simulink model "basic_pid_impedance"  (R2015a)
settings: Solver=ode45  StartTime=0.0  StopTime=10.0  RelTol=1e-3
values from neighbouring files (symbols this model uses):
  pid_imp_Kd = 2    [parameters.m]
  pid_imp_Kp = 40    [parameters.m]
  tau_max = 5    [parameters.m]
undefined symbols (not defined in the file or in its folder): pid
libraries: simulink x1
settings Model: Creator=preston  LastModifiedBy=Nathan

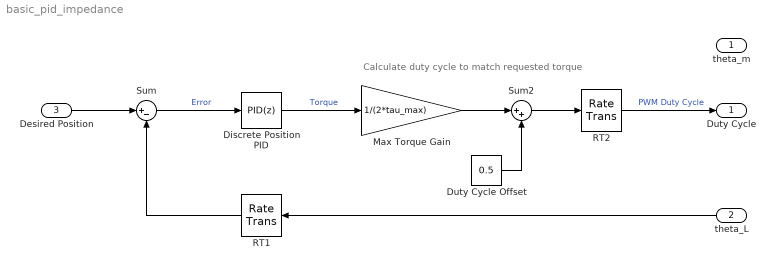
== system basic_pid_impedance ==
  note: Calculate duty cycle to match requested torque
  theta_m : Inport
  theta_L : Inport  Port=2
  Desired Position : Inport  Port=3
  Discrete Position PID : simulink/Continuous/PID Controller  Controller=PID  TimeDomain=Discrete-time  SampleTime=-1  IntegratorMethod=Backward Euler  FilterMethod=Forward Euler  Form=Parallel  UseFilter=off  ControllerParametersSource=internal  P=pid_imp_Kp  I=0  D=pid_imp_Kd  N=pid.N  InitialConditionSource=internal  InitialConditionForIntegrator=0  InitialConditionForFilter=0  ExternalReset=none  LimitOutput=on  UpperSaturationLimit=tau_max  LowerSaturationLimit=-tau_max  LinearizeAsGain=off  AntiWindupMode=none  Kb=1  TrackingMode=off  Kt=1  PParamMin=[]  PParamMax=[]  IParamMin=[]  IParamMax=[]  DParamMin=[]  DParamMax=[]  NParamMin=[]  NParamMax=[]  KbParamMin=[]  KbParamMax=[]  KtParamMin=[]  KtParamMax=[]  POutMin=[]  POutMax=[]  IOutMin=[]  IOutMax=[]  DOutMin=[]  DOutMax=[]  NOutMin=[]  NOutMax=[]  KbOutMin=[]  KbOutMax=[]  KtOutMin=[]  KtOutMax=[]  IntegratorOutMin=[]  IntegratorOutMax=[]  FilterOutMin=[]  FilterOutMax=[]  SumOutMin=[]  SumOutMax=[]  SumI1OutMin=[]  SumI1OutMax=[]  SumI2OutMin=[]  SumI2OutMax=[]  SumI3OutMin=[]  SumI3OutMax=[]  SumDOutMin=[]  SumDOutMax=[]  SaturationOutMin=[]  SaturationOutMax=[]  IntegratorContinuousStateAttributes=''  IntegratorStateMustResolveToSignalObject=off  IntegratorRTWStateStorageClass=Auto  FilterContinuousStateAttributes=''  FilterStateMustResolveToSignalObject=off  FilterRTWStateStorageClass=Auto  DifferentiatorICPrevScaledInput=0  DifferentiatorOutMin=[]  DifferentiatorOutMax=[]
  Duty Cycle Offset : Constant  Value=0.5
  Max Torque Gain : Gain  Gain=1/(2*tau_max)
  RT1 : RateTransition  OutPortSampleTime=T_sample_control
  RT2 : RateTransition
  Sum : Sum  Inputs=|+-
  Sum2 : Sum  Inputs=|++
  "Duty Cycle " : Outport
  wires:
  Discrete Position PID/1 -> Max Torque Gain/1  "Torque"
  Sum/1 -> Discrete Position PID/1  "Error"
  RT1/1 -> Sum/2
  RT2/1 -> "Duty Cycle "/1  "PWM Duty Cycle"
  theta_L/1 -> RT1/1
  Desired Position/1 -> Sum/1
  Max Torque Gain/1 -> Sum2/1
  Sum2/1 -> RT2/1
  Duty Cycle Offset/1 -> Sum2/2
